simulink library "DYN_AERO"  (Simulink 8.8)
settings: Solver=ode45  StartTime=0.0  StopTime=10.0  RelTol=1e-3  EnableMultiTasking=on
undefined symbols (not defined in the file): DYN_SC_par
libraries: LIB_ROT x4, LIB_DYN x1, LIB_ENV x1
settings Model: Creator=alger  LastModifiedBy=alger

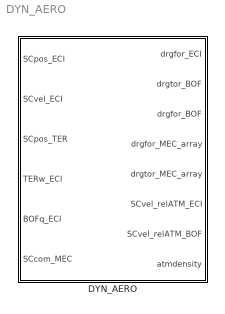
== system DYN_AERO ==
  DYN_AERO : Subsystem

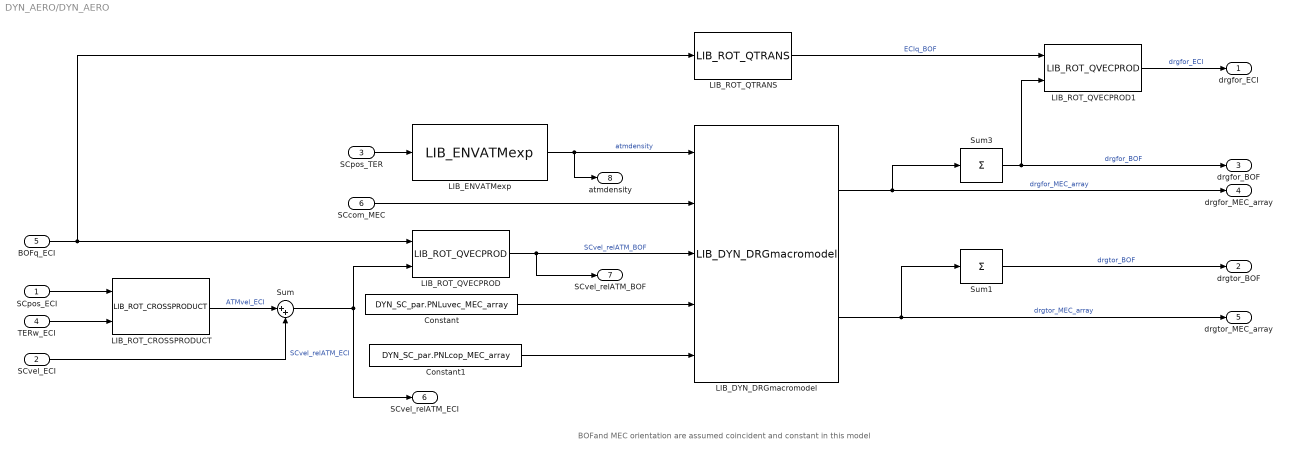
== system DYN_AERO/DYN_AERO ==
  note: BOFand MEC orientation are assumed coincident and constant in this model
  SCpos_ECI : Inport  PortDimensions=3  LockScale=on
  SCvel_ECI : Inport  Port=2  PortDimensions=3  LockScale=on
  SCpos_TER : Inport  Port=3  PortDimensions=3  LockScale=on
  TERw_ECI : Inport  Port=4  PortDimensions=3  LockScale=on
  BOFq_ECI : Inport  Port=5  PortDimensions=4  LockScale=on
  SCcom_MEC : Inport  Port=6  PortDimensions=3  LockScale=on
  Constant : Constant  Value=DYN_SC_par.PNLuvec_MEC_array
  Constant1 : Constant  Value=DYN_SC_par.PNLcop_MEC_array
  "LIB_DYN_DRGmacromodel " : LIB_DYN/LIB_DYN_DRGmacromodel   N=DYN_SC_par.num_panels  pnlarea_array=DYN_SC_par.PNLarea_array  pnlcd_array=DYN_SC_par.PNLcd_array
  LIB_ENVATMexp : LIB_ENV/LIB_ENVATMexp  rho_ref=DYN_AERO_par.rho_REF  height_ref=DYN_AERO_par.H_REF  scale_ref=DYN_AERO_par.scale_REF
  LIB_ROT_CROSSPRODUCT : LIB_ROT/LIB_ROT_CROSSPRODUCT
  LIB_ROT_QTRANS : LIB_ROT/LIB_ROT_QTRANS
  LIB_ROT_QVECPROD : LIB_ROT/LIB_ROT_QVECPROD
  LIB_ROT_QVECPROD1 : LIB_ROT/LIB_ROT_QVECPROD
  Sum : Sum  Inputs=|++
  Sum1 : Sum  Inputs=+  CollapseMode=Specified dimension  CollapseDim=2
  Sum3 : Sum  Inputs=+  CollapseMode=Specified dimension  CollapseDim=2
  drgfor_ECI : Outport  PortDimensions=3
  drgtor_BOF : Outport  Port=2  PortDimensions=3
  drgfor_BOF : Outport  Port=3  PortDimensions=3
  drgfor_MEC_array : Outport  Port=4
  drgtor_MEC_array : Outport  Port=5
  SCvel_relATM_ECI : Outport  Port=6  PortDimensions=3
  SCvel_relATM_BOF : Outport  Port=7  PortDimensions=3
  atmdensity : Outport  Port=8  PortDimensions=1
  wires:
  SCpos_TER/1 -> LIB_ENVATMexp/1
  SCpos_ECI/1 -> LIB_ROT_CROSSPRODUCT/1
  TERw_ECI/1 -> LIB_ROT_CROSSPRODUCT/2
  LIB_ROT_CROSSPRODUCT/1 -> Sum/1  "ATMvel_ECI"
  SCvel_ECI/1 -> Sum/2
  Sum/1 -> LIB_ROT_QVECPROD/2, SCvel_relATM_ECI/1  "SCvel_relATM_ECI"
  BOFq_ECI/1 -> LIB_ROT_QVECPROD/1, LIB_ROT_QTRANS/1
  LIB_ENVATMexp/1 -> atmdensity/1, "LIB_DYN_DRGmacromodel "/1  "atmdensity"
  LIB_ROT_QVECPROD/1 -> SCvel_relATM_BOF/1, "LIB_DYN_DRGmacromodel "/3  "SCvel_relATM_BOF"
  "LIB_DYN_DRGmacromodel "/1 -> drgfor_MEC_array/1, Sum3/1  "drgfor_MEC_array"
  SCcom_MEC/1 -> "LIB_DYN_DRGmacromodel "/2
  Constant/1 -> "LIB_DYN_DRGmacromodel "/4
  Constant1/1 -> "LIB_DYN_DRGmacromodel "/5
  Sum3/1 -> LIB_ROT_QVECPROD1/2, drgfor_BOF/1  "drgfor_BOF"
  Sum1/1 -> drgtor_BOF/1  "drgtor_BOF"
  "LIB_DYN_DRGmacromodel "/2 -> Sum1/1, drgtor_MEC_array/1  "drgtor_MEC_array"
  LIB_ROT_QVECPROD1/1 -> drgfor_ECI/1  "drgfor_ECI"
  LIB_ROT_QTRANS/1 -> LIB_ROT_QVECPROD1/1  "ECIq_BOF"
